simulink model "TwinRotor_G1"  (Simulink 7.2)
settings: Solver=ode1  SolverMode=SingleTasking  StartTime=0.0  StopTime=inf  FixedStep=0.05  RelTol=1e-3
values from neighbouring files (symbols this model uses):
  Kd_tr = 0.01    [def_pid.m]
  Ki_mr = 0.2    [def_pid.m]
  Ki_tr = 0.01    [def_pid.m]
  Kp_mr = 0.05    [def_pid.m]
  Kp_tr = 0.01    [def_pid.m]
libraries: simulink x2, RT x1
settings Model: Creator=Tomás  LastModifiedBy=pdoren
settings DataIOCC: SignalLoggingName=sigsOut
settings OptimizationCC: ExpressionDepthLimit=128  InitFltsAndDblsToZero=on
settings DebuggingCC: SaveWithParameterizedLinksMsg=none  SignalResolutionControl=TryResolveAllWithWarning  SolverPrmCheckMsg=none  MultiTaskDSMMsg=warning  MultiTaskCondExecSysMsg=none  StateNameClashWarn=none  StrictBusMsg=None
settings HardwareCC: TargetIntDivRoundTo=Zero  TargetEndianess=LittleEndian  TargetWordSize=64  TargetHWDeviceType=MATLAB Host  ProdEqTarget=off
settings CodeAppCC: CustomSymbolStrType=$N$R$M_T
settings GRTTargetCC: TargetFcnLib=ansi_tfl_tmw.mat  TargetFunctionLibrary=C89/C90 (ANSI)

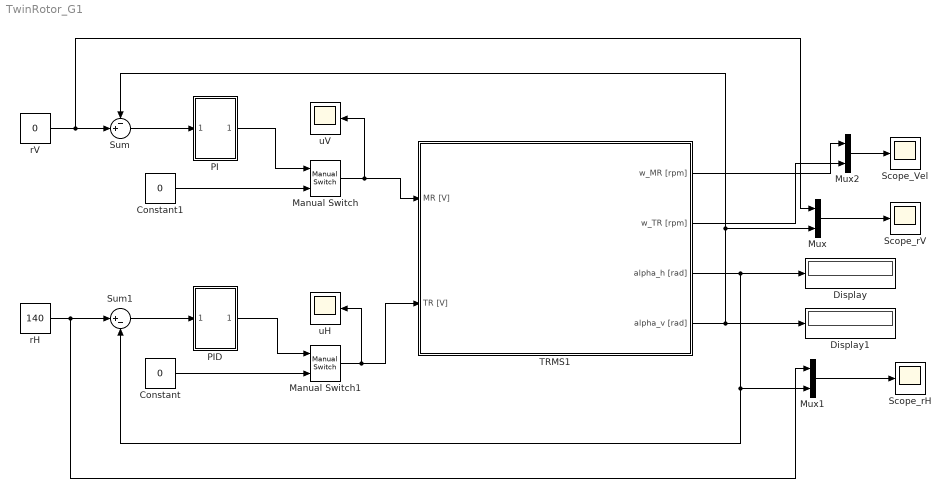
== system TwinRotor_G1 ==
  Constant : Constant  Value=0
  Constant1 : Constant  Value=0
  Display : Display
  Display1 : Display
  Manual Switch : simulink/Signal Routing/Manual Switch  sw=1  action=0  varsize=off
  Manual Switch1 : simulink/Signal Routing/Manual Switch  sw=1  action=0  varsize=off
  Mux : Mux  Inputs=2
  Mux1 : Mux  Inputs=2
  Mux2 : Mux  Inputs=2
  PI : Subsystem
  PID : Subsystem
  Scope_Vel : Scope
      settings: TimeRange=auto  MaxDataPoints=5000  SaveName=Velocidad  YMin=-0.125  YMax=6.125  SampleTime=-1  DataFormat=Array
  Scope_rH : Scope
      settings: TimeRange=auto  MaxDataPoints=5000  SaveName=rH  YMin=107.5  YMax=147.5  SampleTime=-1  DataFormat=Array
  Scope_rV : Scope
      settings: TimeRange=auto  MaxDataPoints=5000  SaveName=rV  YMin=-40  YMax=10  SampleTime=-1  DataFormat=Array
  Sum : Sum  Inputs=-+|
  Sum1 : Sum  Inputs=|+-
  TRMS1 : Subsystem  mask{Ts=0.05, bias_h=0, bias_v=0, max_mr=20, max_tr=15}
      mask prompts: Ts "Tiempo de Muestreo"; bias_h "bias alpha_h"; bias_v "bias alpha_v"; max_mr "voltaje MR [V]"; max_tr "voltaje TR [V]"
      mask Display:
      | image(imread('Imagenes/Copter.png'))
      | 
      | port_label('output', 1, 'w_MR [rpm]')
      | port_label('output', 2, 'w_TR [rpm]')
      | port_label('output', 3, 'alpha_h [deg]')
      | port_label('output', 4, 'alpha_v [deg]')
      | port_label('input', 1, 'MR [V]')
      | port_label('input', 2, 'TR [V]')
  rH : Constant  Value=140
  rV : Constant  Value=0
  uH : Scope
      settings: TimeRange=auto  MaxDataPoints=5000  SaveName=uH  YMin=-1  YMax=1  SampleTime=-1  DataFormat=Array
  uV : Scope
      settings: TimeRange=auto  MaxDataPoints=5000  SaveName=uV  YMin=-207.5  YMax=-167.5  SampleTime=-1  DataFormat=Array
  wires:
  TRMS1/4(alpha_v [rad]) -> Display1/1, Mux/2, Sum/1
  TRMS1/3(alpha_h [rad]) -> Display/1, Mux1/2, Sum1/2
  PI/1(Out1) -> Manual Switch/1
  PID/1(Out1) -> Manual Switch1/1
  Constant/1 -> Manual Switch1/2
  Constant1/1 -> Manual Switch/2
  Sum/1 -> PI/1(In1)
  Sum1/1 -> PID/1(In1)
  Manual Switch/1 -> uV/1, TRMS1/1(MR [V])
  Manual Switch1/1 -> uH/1, TRMS1/2(TR [V])
  rV/1 -> Sum/2, Mux/1
  rH/1 -> Sum1/1, Mux1/1
  Mux2/1 -> Scope_Vel/1
  Mux/1 -> Scope_rV/1
  Mux1/1 -> Scope_rH/1
  TRMS1/1(w_MR [rpm]) -> Mux2/1
  TRMS1/2(w_TR [rpm]) -> Mux2/2

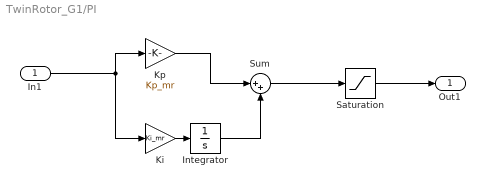
== system TwinRotor_G1/PI ==
  In1 : Inport
  Integrator : Integrator
  Ki : Gain  Gain=Ki_mr
  Kp : Gain  Gain=Kp_mr
  Saturation : Saturate  UpperLimit=20  LowerLimit=0
  Sum : Sum  Inputs=|++
  Out1 : Outport
  wires:
  In1/1 -> Ki/1, Kp/1
  Kp/1 -> Sum/1
  Integrator/1 -> Sum/2
  Ki/1 -> Integrator/1
  Sum/1 -> Saturation/1
  Saturation/1 -> Out1/1

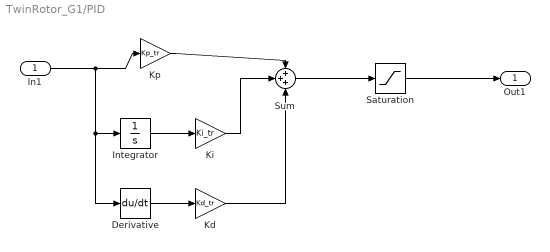
== system TwinRotor_G1/PID ==
  In1 : Inport
  Derivative : Derivative
  Integrator : Integrator
  Kd : Gain  Gain=Kd_tr
  Ki : Gain  Gain=Ki_tr
  Kp : Gain  Gain=Kp_tr
  Saturation : Saturate  UpperLimit=5  LowerLimit=-5
  Sum : Sum  Inputs=+++
  Out1 : Outport
  wires:
  In1/1 -> Kp/1, Integrator/1, Derivative/1
  Kp/1 -> Sum/1
  Sum/1 -> Saturation/1
  Saturation/1 -> Out1/1
  Integrator/1 -> Ki/1
  Ki/1 -> Sum/2
  Derivative/1 -> Kd/1
  Kd/1 -> Sum/3

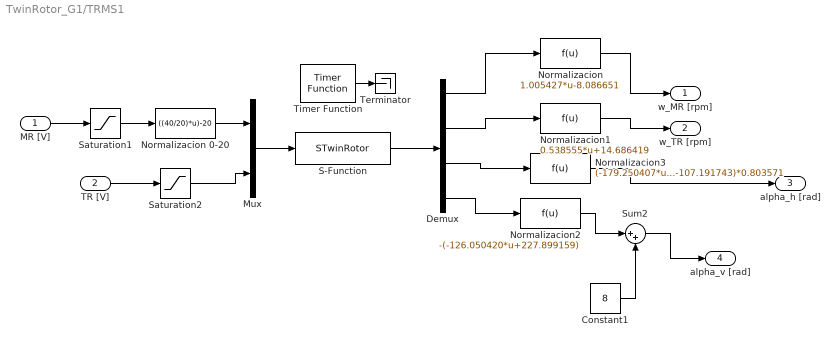
== system TwinRotor_G1/TRMS1 ==
  MR [V] : Inport
  TR [V] : Inport  Port=2
  Constant1 : Constant  Value=8
  Demux : Demux
  Mux : Mux  Inputs=2
  Normalizacion : Fcn  Expr=1.005427*u-8.086651
  Normalizacion 0-20 : Fcn  Expr=((40/20)*u)-20
  Normalizacion1 : Fcn  Expr=0.538555*u+14.686419
  Normalizacion2 : Fcn  Expr=-(-126.050420*u+227.899159)
  Normalizacion3 : Fcn  Expr=(-179.250407*u-107.191743)*0.803571
  S-Function : S-Function  FunctionName=STwinRotor  Parameters=Ts,bias_h,bias_v,max_mr,max_tr  SFunctionDeploymentMode=off  EnableBusSupport=off
  Saturation1 : Saturate  UpperLimit=20  LowerLimit=0
  Saturation2 : Saturate  UpperLimit=5  LowerLimit=-5
  Sum2 : Sum  Inputs=|++
  Terminator : Terminator
  Timer Function : RT/Timer Function  Priority=1234246656  step=50  priority=HIGH  ThPriority=TIME CRITICAL
  w_MR [rpm] : Outport
  w_TR [rpm] : Outport  Port=2
  alpha_h [rad] : Outport  Port=3
  alpha_v [rad] : Outport  Port=4
  wires:
  Constant1/1 -> Sum2/2
  Sum2/1 -> alpha_v [rad]/1
  Normalizacion2/1 -> Sum2/1
  Saturation2/1 -> Mux/2
  Saturation1/1 -> Normalizacion 0-20/1
  Normalizacion3/1 -> alpha_h [rad]/1
  Demux/3 -> Normalizacion3/1
  Demux/4 -> Normalizacion2/1
  Demux/2 -> Normalizacion1/1
  Normalizacion1/1 -> w_TR [rpm]/1
  Demux/1 -> Normalizacion/1
  Normalizacion/1 -> w_MR [rpm]/1
  MR [V]/1 -> Saturation1/1
  Normalizacion 0-20/1 -> Mux/1
  S-Function/1 -> Demux/1
  Mux/1 -> S-Function/1
  TR [V]/1 -> Saturation2/1
  Timer Function/1 -> Terminator/1
